simulink model "two_parallel_full_model_simscape"  (R2023b)
settings: Solver=ode1be  StartTime=0.0  StopTime=simlength  FixedStep=ts_sim  MaxStep=ts_sim
undefined symbols (not defined in the file): fclock, fPWM_INV, fPWM_ZVS, gate_nominal_voltage, I_FS, Iout_dc_nom, ki_i_inv, ki_i_zvs, ki_v_inv, ki_v_zvs, kp_i_inv, kp_i_zvs, kp_v_inv, kp_v_zvs, LFi_dc, LFu_ac, magnitude, n10, omega_grid, RCFu_dc, RLFi_dc, RLFu_ac, tc, Tc, tPWM_ZVS, ts_afe, ts_inv, ts_zvs, ugrid_factor, Ugrid_phase_normalization_factor, un_eta_pu, un_xi_pu, up_xi_pu, v1_trafo, v2_trafo, V_FS, Vout_dc_nom
libraries: fl_lib x142, nesl_utility x55, single_phase_transformer_lib x4
(part 2 of 4)

== system two_parallel_full_model_simscape/load/single_phase_ui_measure ==
  Bus Creator : BusCreator  Inputs=2
  Bus Creator1 : BusCreator  Inputs=2
  Current Sensor : fl_lib/Electrical/Electrical Sensors/Current Sensor
  Selector : Selector  InputPortWidth=2  IndexOptions=Index vector (dialog)  Indices=2  OutputSizes=1
  Selector1 : Selector  InputPortWidth=2  IndexOptions=Index vector (dialog)  Indices=1  OutputSizes=1
  To Workspace1 : ToWorkspace  VariableName=load_current_sim  SampleTime=tc
      settings: MaxDataPoints=Nc
  To Workspace2 : ToWorkspace  VariableName=load_voltage_sim  SampleTime=tc
      settings: MaxDataPoints=Nc
  Voltage Sensor : fl_lib/Electrical/Electrical Sensors/Voltage Sensor
  idc/udc zvs modA : Scope  NumInputPorts=2
  iload/imod1/imod2 : Scope  NumInputPorts=2
  iph : nesl_utility/PS-Simulink Converter  PhysicalDomain=network_engine_domain  SubClassName=ps_output  LeftPortType=input  RightPortType=output  PseudoPeriodic=off  Frequencies=[]  VectorFormat=1-D array  Unit=A  AffineConversion=off
  uph : nesl_utility/PS-Simulink Converter  PhysicalDomain=network_engine_domain  SubClassName=ps_output  LeftPortType=input  RightPortType=output  PseudoPeriodic=off  Frequencies=[]  VectorFormat=1-D array  Unit=V  AffineConversion=off
  Ua : PMIOPort  Side=Left
  ua : PMIOPort  Port=2  Side=Right
  Ub : PMIOPort  Port=3  Side=Left
  ub : PMIOPort  Port=4  Side=Right
  tag scope: load_current=global, load_voltage=global
  wires:
  [load_current] -> idc/udc zvs modA/1
  [load_voltage] -> idc/udc zvs modA/2
  Selector1/1 -> [load_current]
  Selector/1 -> [load_voltage]
  Bus Creator/1 -> Selector/1, Selector1/1  "ui_data"
  iph/1 -> Bus Creator/1  "iph"
  uph/1 -> Bus Creator/2  "uph"
  [load_current] -> To Workspace1/1
  [load_voltage] -> To Workspace2/1
  [load_current] -> iload/imod1/imod2/1  "i_load"
  [inverter_current_output_modA] -> Bus Creator1/1  "i_modA"
  [inverter_current_output_modB] -> Bus Creator1/2  "i_modB"
  Bus Creator1/1 -> iload/imod1/imod2/2  "i_modAB"
  connections:
  iph/LConn1 -- Current Sensor/RConn1
  Voltage Sensor/LConn1 -- Current Sensor/LConn1 -- Ua/RConn1
  Current Sensor/RConn2 -- ua/RConn1
  Voltage Sensor/RConn1 -- uph/LConn1
  Voltage Sensor/RConn2 -- Ub/RConn1 -- ub/RConn1

== system two_parallel_full_model_simscape/zvs_modA/dc//dc with galvanic isolation ==
  gate_commands : Inport
  CFu_dc : fl_lib/Electrical/Electrical Elements/Capacitor  c=CFu_dc F  r=RCFu_dc_internal Ohm  g=0 1/Ohm  i_specify=off  i_priority=None  i=0 A  i_nominal_specify=off  i_nominal_unit=A  i_nominal_value=1  v_specify=off  v_priority=None  v=0 V  v_nominal_specify=off  v_nominal_unit=V  v_nominal_value=1  vc_specify=off  vc_priority=High  vc=0 V  vc_nominal_specify=off  vc_nominal_unit=V  vc_nominal_value=1
  Electrical Reference : fl_lib/Electrical/Electrical Elements/Electrical Reference
  RCFu_dc : fl_lib/Electrical/Electrical Elements/Resistor  R=RCFu_dc Ohm  i_specify=off  i_priority=None  i=0 A  i_nominal_specify=off  i_nominal_unit=A  i_nominal_value=1  v_specify=off  v_priority=None  v=0 V  v_nominal_specify=off  v_nominal_unit=V  v_nominal_value=1
  blider1 : fl_lib/Electrical/Electrical Elements/Resistor  R=1e4 Ohm  i_specify=off  i_priority=None  i=0 A  i_nominal_specify=off  i_nominal_unit=A  i_nominal_value=1  v_specify=off  v_priority=None  v=0 V  v_nominal_specify=off  v_nominal_unit=V  v_nominal_value=1
  blider2 : fl_lib/Electrical/Electrical Elements/Resistor  R=1e4 Ohm  i_specify=off  i_priority=None  i=0 A  i_nominal_specify=off  i_nominal_unit=A  i_nominal_value=1  v_specify=off  v_priority=None  v=0 V  v_nominal_specify=off  v_nominal_unit=V  v_nominal_value=1
  stage-1 : Subsystem
      settings: PortSchema="{\"entries\":[{\"content\":{\"sides\":[{\"content\":{\"connectorIds\":[\"LConn1\",\"LConn2\"]},\"type\":\"ConnectorPlacement.EquallySpacedRectSide\",\"uuid\":\"c872503a-61af-4937-bdf2-4de4f8645573\"},{\"content\":{\"connectorIds\":[\"RConn1\",\"RConn2\"],\"side\":\"RIGHT\"},\"type\":\"ConnectorPlacement.EquallySpacedRectSide\",\"uuid\":\"3b83f060-86a2-4569-84b5-d9f7c0485347\"},{\"content\":{\"connectorIds\":[\"In1\"],\"side\":\"TOP\"},\"type\":\"ConnectorPlacement.EquallySpacedRectSide\",\"uuid\":\"bf191d46-ce71-4d15-9dd0-24cc57253577\"}]},\"type\":\"ConnectorPlacement.EquallySpacedConnector\",\"uuid\":\"1b28ceee-25d0-45ae-a3c4-c2563f0d63ba\"}],\"packageUris\":[\"http://schema.mathworks.com/mf0/Connector/R2020b\"],\"version\":\"1.0\"}"
  stage-2 : Subsystem
  Udc(+) : PMIOPort  Side=Left
  udc(+) : PMIOPort  Port=2  Side=Right
  Udc(-) : PMIOPort  Port=3  Side=Left
  udc(-) : PMIOPort  Port=4  Side=Right
  wires:
  gate_commands/1 -> stage-1/1(gate_commands)
  connections:
  stage-2/LConn1 -- stage-1/LConn1
  stage-2/LConn2 -- stage-1/LConn2
  stage-1/RConn1 -- Udc(+)/RConn1
  stage-1/RConn2 -- Udc(-)/RConn1
  CFu_dc/RConn1 -- RCFu_dc/RConn1 -- stage-2/RConn2 -- blider2/RConn1 -- udc(-)/RConn1
  blider2/LConn1 -- blider1/RConn1 -- Electrical Reference/LConn1
  RCFu_dc/LConn1 -- udc(+)/RConn1 -- blider1/LConn1 -- CFu_dc/LConn1 -- stage-2/RConn1

== system two_parallel_full_model_simscape/zvs_modA/grid_rectifier ==
  CFi : fl_lib/Electrical/Electrical Elements/Capacitor  c=CFi_dc F  r=RCFi_dc Ohm  g=0 1/Ohm  i_specify=off  i_priority=None  i=0 A  i_nominal_specify=off  i_nominal_unit=A  i_nominal_value=1  v_specify=off  v_priority=None  v=0 V  v_nominal_specify=off  v_nominal_unit=V  v_nominal_value=1  vc_specify=off  vc_priority=High  vc=0 V  vc_nominal_specify=off  vc_nominal_unit=V  vc_nominal_value=1
  LFi_1 : fl_lib/Electrical/Electrical Elements/Inductor  l=LFi_dc/2 H  r=RLFi_dc/2 Ohm  g=1e-9 1/Ohm  i_specify=on  i_priority=High  i=0 A  i_nominal_specify=off  i_nominal_unit=A  i_nominal_value=1  v_specify=off  v_priority=None  v=0 V  v_nominal_specify=off  v_nominal_unit=V  v_nominal_value=1  i_L_specify=off  i_L_priority=High  i_L=0 A  i_L_nominal_specify=off  i_L_nominal_unit=A  i_L_nominal_value=1
  LFi_2 : fl_lib/Electrical/Electrical Elements/Inductor  l=LFi_dc/2 H  r=RLFi_dc/2 Ohm  g=1e-9 1/Ohm  i_specify=on  i_priority=High  i=0 A  i_nominal_specify=off  i_nominal_unit=A  i_nominal_value=1  v_specify=off  v_priority=None  v=0 V  v_nominal_specify=off  v_nominal_unit=V  v_nominal_value=1  i_L_specify=off  i_L_priority=High  i_L=0 A  i_L_nominal_specify=off  i_L_nominal_unit=A  i_L_nominal_value=1
  three-phase-rectifier : Subsystem
  rectifier_udc(+) : PMIOPort  Side=Right
  ua : PMIOPort  Port=2  Side=Left
  ub : PMIOPort  Port=3  Side=Left
  uc : PMIOPort  Port=4  Side=Left
  rectifier_udc(-) : PMIOPort  Port=5  Side=Right
  connections:
  LFi_1/RConn1 -- rectifier_udc(+)/RConn1 -- CFi/LConn1
  LFi_2/LConn1 -- rectifier_udc(-)/RConn1 -- CFi/RConn1
  LFi_1/LConn1 -- three-phase-rectifier/RConn1
  three-phase-rectifier/LConn1 -- ua/RConn1
  three-phase-rectifier/LConn2 -- ub/RConn1
  three-phase-rectifier/LConn3 -- uc/RConn1
  LFi_2/RConn1 -- three-phase-rectifier/RConn2

== system two_parallel_full_model_simscape/zvs_modA/measurment ==
  To Workspace10 : ToWorkspace  VariableName=vi_CFu_ac_modA_sim  SampleTime=Tc
      settings: MaxDataPoints=Nc
  To Workspace11 : ToWorkspace  VariableName=vi_LFu_ac_modA_sim  SampleTime=Tc
      settings: MaxDataPoints=Nc
  To Workspace12 : ToWorkspace  VariableName=vi_LFi_dc_modA_sim  SampleTime=Tc
      settings: MaxDataPoints=Nc
  To Workspace13 : ToWorkspace  VariableName=vi_Ls_modA_sim  SampleTime=Tc
      settings: MaxDataPoints=Nc
  To Workspace14 : ToWorkspace  VariableName=vi_CFi_dc_modA_sim  SampleTime=Tc
      settings: MaxDataPoints=Nc
  To Workspace15 : ToWorkspace  VariableName=i_d_rect_modA_sim  SampleTime=Tc
      settings: MaxDataPoints=Nc
  To Workspace2 : ToWorkspace  VariableName=vi_RCFu_dc_modA_sim  SampleTime=Tc
      settings: MaxDataPoints=Nc
  To Workspace3 : ToWorkspace  VariableName=vi_LFu_dc_modA_sim  SampleTime=Tc
      settings: MaxDataPoints=Nc
  To Workspace4 : ToWorkspace  VariableName=vi_Cs_modA_sim  SampleTime=Tc
      settings: MaxDataPoints=Nc
  To Workspace5 : ToWorkspace  VariableName=vi_load_modA_sim  SampleTime=Tc
      settings: MaxDataPoints=Nc
  To Workspace6 : ToWorkspace  VariableName=vi_CFu_dc_modA_sim  SampleTime=Tc
      settings: MaxDataPoints=Nc
  To Workspace7 : ToWorkspace  VariableName=vdc_in_modA_sim  SampleTime=Tc
      settings: MaxDataPoints=Nc
  To Workspace8 : ToWorkspace  VariableName=Isnubber_H_modA_sim  SampleTime=Tc
      settings: MaxDataPoints=Nc
  To Workspace9 : ToWorkspace  VariableName=Isnubber_Rect1_modA_sim  SampleTime=Tc
      settings: MaxDataPoints=Nc

== system two_parallel_full_model_simscape/zvs_modA/single_phase_ui_measure ==
  Bus Creator : BusCreator  Inputs=2
  Current Sensor : fl_lib/Electrical/Electrical Sensors/Current Sensor
  Selector : Selector  InputPortWidth=2  IndexOptions=Index vector (dialog)  Indices=2  OutputSizes=1
  Selector1 : Selector  InputPortWidth=2  IndexOptions=Index vector (dialog)  Indices=1  OutputSizes=1
  To Workspace1 : ToWorkspace  VariableName=zvs_current_output_modA_sim  SampleTime=tc
      settings: MaxDataPoints=Nc
  To Workspace2 : ToWorkspace  VariableName=zvs_voltage_output_modA_sim  SampleTime=tc
      settings: MaxDataPoints=Nc
  Voltage Sensor : fl_lib/Electrical/Electrical Sensors/Voltage Sensor
  idc/udc zvs modA : Scope  NumInputPorts=2
  iph : nesl_utility/PS-Simulink Converter  PhysicalDomain=network_engine_domain  SubClassName=ps_output  LeftPortType=input  RightPortType=output  PseudoPeriodic=off  Frequencies=[]  VectorFormat=1-D array  Unit=A  AffineConversion=off
  uph : nesl_utility/PS-Simulink Converter  PhysicalDomain=network_engine_domain  SubClassName=ps_output  LeftPortType=input  RightPortType=output  PseudoPeriodic=off  Frequencies=[]  VectorFormat=1-D array  Unit=V  AffineConversion=off
  Udc(+) : PMIOPort  Side=Left
  udc(+) : PMIOPort  Port=2  Side=Right
  Udc(-) : PMIOPort  Port=3  Side=Left
  udc(-) : PMIOPort  Port=4  Side=Right
  tag scope: zvs_current_output_modA=global, zvs_voltage_output_modA=global
  wires:
  [zvs_current_output_modA] -> idc/udc zvs modA/1  "zvs_current_output_modA"
  [zvs_voltage_output_modA] -> idc/udc zvs modA/2  "zvs_voltage_output_modA"
  Selector1/1 -> [zvs_current_output_modA]
  Selector/1 -> [zvs_voltage_output_modA]
  Bus Creator/1 -> Selector/1, Selector1/1  "ui_data"
  iph/1 -> Bus Creator/1  "iph"
  uph/1 -> Bus Creator/2  "uph"
  [zvs_current_output_modA] -> To Workspace1/1
  [zvs_voltage_output_modA] -> To Workspace2/1
  connections:
  iph/LConn1 -- Current Sensor/RConn1
  Voltage Sensor/LConn1 -- Current Sensor/LConn1 -- Udc(+)/RConn1
  Current Sensor/RConn2 -- udc(+)/RConn1
  Voltage Sensor/RConn1 -- uph/LConn1
  Voltage Sensor/RConn2 -- Udc(-)/RConn1 -- udc(-)/RConn1

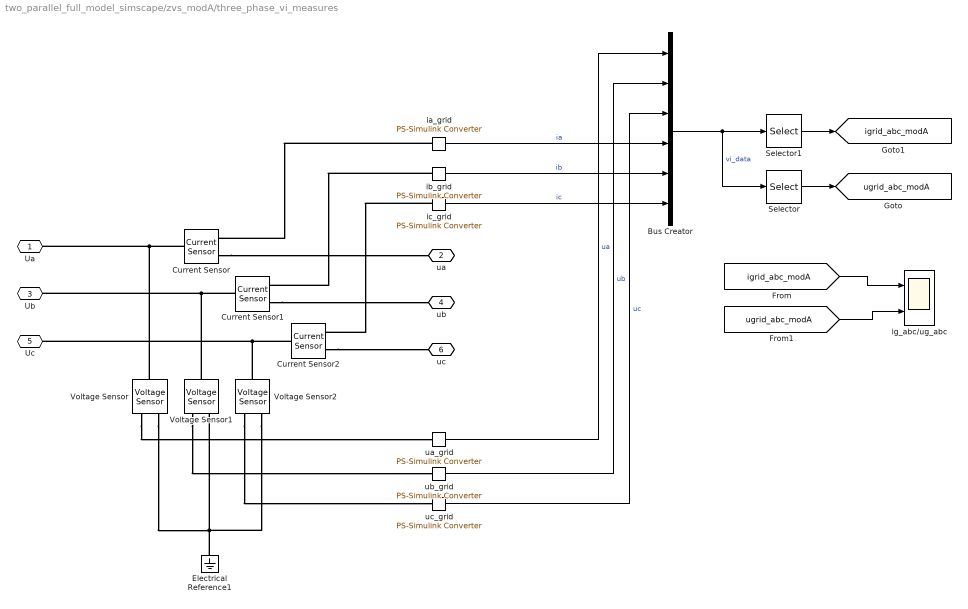
== system two_parallel_full_model_simscape/zvs_modA/three_phase_vi_measures ==
  Bus Creator : BusCreator  Inputs=6
  Current Sensor : fl_lib/Electrical/Electrical Sensors/Current Sensor
  Current Sensor1 : fl_lib/Electrical/Electrical Sensors/Current Sensor
  Current Sensor2 : fl_lib/Electrical/Electrical Sensors/Current Sensor
  Electrical Reference1 : fl_lib/Electrical/Electrical Elements/Electrical Reference
  Selector : Selector  InputPortWidth=6  IndexOptions=Index vector (dialog)  Indices=[1 2 3]  OutputSizes=1
  Selector1 : Selector  InputPortWidth=6  IndexOptions=Index vector (dialog)  Indices=[4 5 6]  OutputSizes=1
  Voltage Sensor : fl_lib/Electrical/Electrical Sensors/Voltage Sensor
  Voltage Sensor1 : fl_lib/Electrical/Electrical Sensors/Voltage Sensor
  Voltage Sensor2 : fl_lib/Electrical/Electrical Sensors/Voltage Sensor
  ia_grid : nesl_utility/PS-Simulink Converter  PhysicalDomain=network_engine_domain  SubClassName=ps_output  LeftPortType=input  RightPortType=output  PseudoPeriodic=off  Frequencies=[]  VectorFormat=1-D array  Unit=A  AffineConversion=off
  ib_grid : nesl_utility/PS-Simulink Converter  PhysicalDomain=network_engine_domain  SubClassName=ps_output  LeftPortType=input  RightPortType=output  PseudoPeriodic=off  Frequencies=[]  VectorFormat=1-D array  Unit=A  AffineConversion=off
  ic_grid : nesl_utility/PS-Simulink Converter  PhysicalDomain=network_engine_domain  SubClassName=ps_output  LeftPortType=input  RightPortType=output  PseudoPeriodic=off  Frequencies=[]  VectorFormat=1-D array  Unit=A  AffineConversion=off
  ig_abc/ug_abc : Scope  NumInputPorts=2
  ua_grid : nesl_utility/PS-Simulink Converter  PhysicalDomain=network_engine_domain  SubClassName=ps_output  LeftPortType=input  RightPortType=output  PseudoPeriodic=off  Frequencies=[]  VectorFormat=1-D array  Unit=V  AffineConversion=off
  ub_grid : nesl_utility/PS-Simulink Converter  PhysicalDomain=network_engine_domain  SubClassName=ps_output  LeftPortType=input  RightPortType=output  PseudoPeriodic=off  Frequencies=[]  VectorFormat=1-D array  Unit=V  AffineConversion=off
  uc_grid : nesl_utility/PS-Simulink Converter  PhysicalDomain=network_engine_domain  SubClassName=ps_output  LeftPortType=input  RightPortType=output  PseudoPeriodic=off  Frequencies=[]  VectorFormat=1-D array  Unit=V  AffineConversion=off
  Ua : PMIOPort  Side=Left
  ua : PMIOPort  Port=2  Side=Right
  Ub : PMIOPort  Port=3  Side=Left
  ub : PMIOPort  Port=4  Side=Right
  Uc : PMIOPort  Port=5  Side=Left
  uc : PMIOPort  Port=6  Side=Right
  tag scope: igrid_abc_modA=global, ugrid_abc_modA=global
  wires:
  Bus Creator/1 -> Selector1/1, Selector/1  "vi_data"
  Selector/1 -> [ugrid_abc_modA]
  ib_grid/1 -> Bus Creator/5  "ib"
  ia_grid/1 -> Bus Creator/4  "ia"
  ic_grid/1 -> Bus Creator/6  "ic"
  ua_grid/1 -> Bus Creator/1  "ua"
  ub_grid/1 -> Bus Creator/2  "ub"
  uc_grid/1 -> Bus Creator/3  "uc"
  Selector1/1 -> [igrid_abc_modA]
  [ugrid_abc_modA] -> ig_abc/ug_abc/2
  [igrid_abc_modA] -> ig_abc/ug_abc/1
  connections:
  Current Sensor1/LConn1 -- Ub/RConn1 -- Voltage Sensor1/LConn1
  Electrical Reference1/LConn1 -- Voltage Sensor/RConn2 -- Voltage Sensor2/RConn2 -- Voltage Sensor1/RConn2
  Voltage Sensor/RConn1 -- ua_grid/LConn1
  Current Sensor/RConn2 -- ua/RConn1
  Voltage Sensor1/RConn1 -- ub_grid/LConn1
  Voltage Sensor2/LConn1 -- Current Sensor2/LConn1 -- Uc/RConn1
  Current Sensor/LConn1 -- Ua/RConn1 -- Voltage Sensor/LConn1
  Current Sensor1/RConn2 -- ub/RConn1
  Voltage Sensor2/RConn1 -- uc_grid/LConn1
  ib_grid/LConn1 -- Current Sensor1/RConn1
  ia_grid/LConn1 -- Current Sensor/RConn1
  ic_grid/LConn1 -- Current Sensor2/RConn1
  Current Sensor2/RConn2 -- uc/RConn1

== system two_parallel_full_model_simscape/zvs_modA/zvs_ctrl ==
  Bus Creator : BusCreator  Inputs=4
  modulator : Subsystem
  references : Subsystem
  sampling_i_filter1 : Subsystem
  sampling_v_filter1 : Subsystem
  sampling_v_filter2 : Subsystem
  vi ctrl : Subsystem
  gate_commands : Outport
  wires:
  [zvs_voltage_output_modA] -> sampling_v_filter1/1(in)
  [zvs_current_output_modA] -> sampling_i_filter1/1(in)
  vi ctrl/1(phase_displacement) -> modulator/1(phase_displacement)
  sampling_i_filter1/1(out_pu) -> vi ctrl/1(iout)
  sampling_v_filter1/1(out_pu) -> vi ctrl/2(vout)
  sampling_v_filter2/1(out_pu) -> vi ctrl/3(vout_ref)
  references/1(vout_ref) -> sampling_v_filter2/1(in)
  Bus Creator/1 -> gate_commands/1
  modulator/1(gate_Q1) -> Bus Creator/1
  modulator/2(gate_Q2) -> Bus Creator/2
  modulator/3(gate_Q3) -> Bus Creator/3
  modulator/4(gate_Q4) -> Bus Creator/4

== system two_parallel_full_model_simscape/zvs_modB/dc//dc with galvanic isolation ==
  gate_commands : Inport
  CFu_dc : fl_lib/Electrical/Electrical Elements/Capacitor  c=CFu_dc F  r=RCFu_dc_internal Ohm  g=0 1/Ohm  i_specify=off  i_priority=None  i=0 A  i_nominal_specify=off  i_nominal_unit=A  i_nominal_value=1  v_specify=off  v_priority=None  v=0 V  v_nominal_specify=off  v_nominal_unit=V  v_nominal_value=1  vc_specify=off  vc_priority=High  vc=0 V  vc_nominal_specify=off  vc_nominal_unit=V  vc_nominal_value=1
  Electrical Reference : fl_lib/Electrical/Electrical Elements/Electrical Reference
  RCFu_dc : fl_lib/Electrical/Electrical Elements/Resistor  R=RCFu_dc Ohm  i_specify=off  i_priority=None  i=0 A  i_nominal_specify=off  i_nominal_unit=A  i_nominal_value=1  v_specify=off  v_priority=None  v=0 V  v_nominal_specify=off  v_nominal_unit=V  v_nominal_value=1
  blider1 : fl_lib/Electrical/Electrical Elements/Resistor  R=1e4 Ohm  i_specify=off  i_priority=None  i=0 A  i_nominal_specify=off  i_nominal_unit=A  i_nominal_value=1  v_specify=off  v_priority=None  v=0 V  v_nominal_specify=off  v_nominal_unit=V  v_nominal_value=1
  blider2 : fl_lib/Electrical/Electrical Elements/Resistor  R=1e4 Ohm  i_specify=off  i_priority=None  i=0 A  i_nominal_specify=off  i_nominal_unit=A  i_nominal_value=1  v_specify=off  v_priority=None  v=0 V  v_nominal_specify=off  v_nominal_unit=V  v_nominal_value=1
  stage-1 : Subsystem
      settings: PortSchema="{\"entries\":[{\"content\":{\"sides\":[{\"content\":{\"connectorIds\":[\"LConn1\",\"LConn2\"]},\"type\":\"ConnectorPlacement.EquallySpacedRectSide\",\"uuid\":\"c872503a-61af-4937-bdf2-4de4f8645573\"},{\"content\":{\"connectorIds\":[\"RConn1\",\"RConn2\"],\"side\":\"RIGHT\"},\"type\":\"ConnectorPlacement.EquallySpacedRectSide\",\"uuid\":\"3b83f060-86a2-4569-84b5-d9f7c0485347\"},{\"content\":{\"connectorIds\":[\"In1\"],\"side\":\"TOP\"},\"type\":\"ConnectorPlacement.EquallySpacedRectSide\",\"uuid\":\"bf191d46-ce71-4d15-9dd0-24cc57253577\"}]},\"type\":\"ConnectorPlacement.EquallySpacedConnector\",\"uuid\":\"1b28ceee-25d0-45ae-a3c4-c2563f0d63ba\"}],\"packageUris\":[\"http://schema.mathworks.com/mf0/Connector/R2020b\"],\"version\":\"1.0\"}"
  stage-2 : Subsystem
  Udc(+) : PMIOPort  Side=Left
  udc(+) : PMIOPort  Port=2  Side=Right
  Udc(-) : PMIOPort  Port=3  Side=Left
  udc(-) : PMIOPort  Port=4  Side=Right
  wires:
  gate_commands/1 -> stage-1/1(gate_commands)
  connections:
  stage-2/RConn1 -- CFu_dc/LConn1 -- blider1/LConn1 -- udc(+)/RConn1 -- RCFu_dc/LConn1
  Electrical Reference/LConn1 -- blider1/RConn1 -- blider2/LConn1
  udc(-)/RConn1 -- blider2/RConn1 -- stage-2/RConn2 -- RCFu_dc/RConn1 -- CFu_dc/RConn1
  stage-1/RConn2 -- Udc(-)/RConn1
  stage-1/RConn1 -- Udc(+)/RConn1
  stage-2/LConn2 -- stage-1/LConn2
  stage-2/LConn1 -- stage-1/LConn1

== system two_parallel_full_model_simscape/zvs_modB/grid_rectifier ==
  CFi : fl_lib/Electrical/Electrical Elements/Capacitor  c=CFi_dc F  r=RCFi_dc Ohm  g=0 1/Ohm  i_specify=off  i_priority=None  i=0 A  i_nominal_specify=off  i_nominal_unit=A  i_nominal_value=1  v_specify=off  v_priority=None  v=0 V  v_nominal_specify=off  v_nominal_unit=V  v_nominal_value=1  vc_specify=off  vc_priority=High  vc=0 V  vc_nominal_specify=off  vc_nominal_unit=V  vc_nominal_value=1
  LFi_1 : fl_lib/Electrical/Electrical Elements/Inductor  l=LFi_dc/2 H  r=RLFi_dc/2 Ohm  g=1e-9 1/Ohm  i_specify=on  i_priority=High  i=0 A  i_nominal_specify=off  i_nominal_unit=A  i_nominal_value=1  v_specify=off  v_priority=None  v=0 V  v_nominal_specify=off  v_nominal_unit=V  v_nominal_value=1  i_L_specify=off  i_L_priority=High  i_L=0 A  i_L_nominal_specify=off  i_L_nominal_unit=A  i_L_nominal_value=1
  LFi_2 : fl_lib/Electrical/Electrical Elements/Inductor  l=LFi_dc/2 H  r=RLFi_dc/2 Ohm  g=1e-9 1/Ohm  i_specify=on  i_priority=High  i=0 A  i_nominal_specify=off  i_nominal_unit=A  i_nominal_value=1  v_specify=off  v_priority=None  v=0 V  v_nominal_specify=off  v_nominal_unit=V  v_nominal_value=1  i_L_specify=off  i_L_priority=High  i_L=0 A  i_L_nominal_specify=off  i_L_nominal_unit=A  i_L_nominal_value=1
  three-phase-rectifier : Subsystem
  rectifier_udc(+) : PMIOPort  Side=Right
  ua : PMIOPort  Port=2  Side=Left
  ub : PMIOPort  Port=3  Side=Left
  uc : PMIOPort  Port=4  Side=Left
  rectifier_udc(-) : PMIOPort  Port=5  Side=Right
  connections:
  LFi_2/RConn1 -- three-phase-rectifier/RConn2
  three-phase-rectifier/LConn3 -- uc/RConn1
  three-phase-rectifier/LConn2 -- ub/RConn1
  three-phase-rectifier/LConn1 -- ua/RConn1
  LFi_1/LConn1 -- three-phase-rectifier/RConn1
  CFi/RConn1 -- rectifier_udc(-)/RConn1 -- LFi_2/LConn1
  CFi/LConn1 -- rectifier_udc(+)/RConn1 -- LFi_1/RConn1

== system two_parallel_full_model_simscape/zvs_modB/measurment ==
  To Workspace10 : ToWorkspace  VariableName=vi_CFu_ac_modA_sim  SampleTime=Tc
      settings: MaxDataPoints=Nc
  To Workspace11 : ToWorkspace  VariableName=vi_LFu_ac_modA_sim  SampleTime=Tc
      settings: MaxDataPoints=Nc
  To Workspace12 : ToWorkspace  VariableName=vi_LFi_dc_modA_sim  SampleTime=Tc
      settings: MaxDataPoints=Nc
  To Workspace13 : ToWorkspace  VariableName=vi_Ls_modA_sim  SampleTime=Tc
      settings: MaxDataPoints=Nc
  To Workspace14 : ToWorkspace  VariableName=vi_CFi_dc_modA_sim  SampleTime=Tc
      settings: MaxDataPoints=Nc
  To Workspace15 : ToWorkspace  VariableName=i_d_rect_modA_sim  SampleTime=Tc
      settings: MaxDataPoints=Nc
  To Workspace2 : ToWorkspace  VariableName=vi_RCFu_dc_modA_sim  SampleTime=Tc
      settings: MaxDataPoints=Nc
  To Workspace3 : ToWorkspace  VariableName=vi_LFu_dc_modA_sim  SampleTime=Tc
      settings: MaxDataPoints=Nc
  To Workspace4 : ToWorkspace  VariableName=vi_Cs_modA_sim  SampleTime=Tc
      settings: MaxDataPoints=Nc
  To Workspace5 : ToWorkspace  VariableName=vi_load_modA_sim  SampleTime=Tc
      settings: MaxDataPoints=Nc
  To Workspace6 : ToWorkspace  VariableName=vi_CFu_dc_modA_sim  SampleTime=Tc
      settings: MaxDataPoints=Nc
  To Workspace7 : ToWorkspace  VariableName=vdc_in_modA_sim  SampleTime=Tc
      settings: MaxDataPoints=Nc
  To Workspace8 : ToWorkspace  VariableName=Isnubber_H_modA_sim  SampleTime=Tc
      settings: MaxDataPoints=Nc
  To Workspace9 : ToWorkspace  VariableName=Isnubber_Rect1_modA_sim  SampleTime=Tc
      settings: MaxDataPoints=Nc

== system two_parallel_full_model_simscape/zvs_modB/single_phase_ui_measure ==
  Bus Creator : BusCreator  Inputs=2
  Current Sensor : fl_lib/Electrical/Electrical Sensors/Current Sensor
  Selector : Selector  InputPortWidth=2  IndexOptions=Index vector (dialog)  Indices=2  OutputSizes=1
  Selector1 : Selector  InputPortWidth=2  IndexOptions=Index vector (dialog)  Indices=1  OutputSizes=1
  To Workspace1 : ToWorkspace  VariableName=zvs_current_output_modB_sim  SampleTime=tc
      settings: MaxDataPoints=Nc
  To Workspace2 : ToWorkspace  VariableName=zvs_voltage_output_modB_sim  SampleTime=tc
      settings: MaxDataPoints=Nc
  Voltage Sensor : fl_lib/Electrical/Electrical Sensors/Voltage Sensor
  idc/udc zvs modB : Scope  NumInputPorts=2
  iph : nesl_utility/PS-Simulink Converter  PhysicalDomain=network_engine_domain  SubClassName=ps_output  LeftPortType=input  RightPortType=output  PseudoPeriodic=off  Frequencies=[]  VectorFormat=1-D array  Unit=A  AffineConversion=off
  uph : nesl_utility/PS-Simulink Converter  PhysicalDomain=network_engine_domain  SubClassName=ps_output  LeftPortType=input  RightPortType=output  PseudoPeriodic=off  Frequencies=[]  VectorFormat=1-D array  Unit=V  AffineConversion=off
  Udc(+) : PMIOPort  Side=Left
  udc(+) : PMIOPort  Port=2  Side=Right
  Udc(-) : PMIOPort  Port=3  Side=Left
  udc(-) : PMIOPort  Port=4  Side=Right
  tag scope: zvs_current_output_modB=global, zvs_voltage_output_modB=global
  wires:
  [zvs_voltage_output_modB] -> To Workspace2/1
  [zvs_current_output_modB] -> To Workspace1/1
  uph/1 -> Bus Creator/2  "uph"
  iph/1 -> Bus Creator/1  "iph"
  Bus Creator/1 -> Selector1/1, Selector/1  "ui_data"
  Selector/1 -> [zvs_voltage_output_modB]
  Selector1/1 -> [zvs_current_output_modB]
  [zvs_voltage_output_modB] -> idc/udc zvs modB/2  "zvs_voltage_output_modB"
  [zvs_current_output_modB] -> idc/udc zvs modB/1  "zvs_current_output_modB"
  connections:
  udc(-)/RConn1 -- Udc(-)/RConn1 -- Voltage Sensor/RConn2
  Voltage Sensor/RConn1 -- uph/LConn1
  Current Sensor/RConn2 -- udc(+)/RConn1
  Udc(+)/RConn1 -- Current Sensor/LConn1 -- Voltage Sensor/LConn1
  iph/LConn1 -- Current Sensor/RConn1

== system two_parallel_full_model_simscape/zvs_modB/three_phase_vi_measures ==
  Bus Creator : BusCreator  Inputs=6
  Current Sensor : fl_lib/Electrical/Electrical Sensors/Current Sensor
  Current Sensor1 : fl_lib/Electrical/Electrical Sensors/Current Sensor
  Current Sensor2 : fl_lib/Electrical/Electrical Sensors/Current Sensor
  Electrical Reference1 : fl_lib/Electrical/Electrical Elements/Electrical Reference
  Selector : Selector  InputPortWidth=6  IndexOptions=Index vector (dialog)  Indices=[1 2 3]  OutputSizes=1
  Selector1 : Selector  InputPortWidth=6  IndexOptions=Index vector (dialog)  Indices=[4 5 6]  OutputSizes=1
  Voltage Sensor : fl_lib/Electrical/Electrical Sensors/Voltage Sensor
  Voltage Sensor1 : fl_lib/Electrical/Electrical Sensors/Voltage Sensor
  Voltage Sensor2 : fl_lib/Electrical/Electrical Sensors/Voltage Sensor
  ia_grid : nesl_utility/PS-Simulink Converter  PhysicalDomain=network_engine_domain  SubClassName=ps_output  LeftPortType=input  RightPortType=output  PseudoPeriodic=off  Frequencies=[]  VectorFormat=1-D array  Unit=A  AffineConversion=off
  ib_grid : nesl_utility/PS-Simulink Converter  PhysicalDomain=network_engine_domain  SubClassName=ps_output  LeftPortType=input  RightPortType=output  PseudoPeriodic=off  Frequencies=[]  VectorFormat=1-D array  Unit=A  AffineConversion=off
  ic_grid : nesl_utility/PS-Simulink Converter  PhysicalDomain=network_engine_domain  SubClassName=ps_output  LeftPortType=input  RightPortType=output  PseudoPeriodic=off  Frequencies=[]  VectorFormat=1-D array  Unit=A  AffineConversion=off
  ig_abc/ug_abc : Scope  NumInputPorts=2
  ua_grid : nesl_utility/PS-Simulink Converter  PhysicalDomain=network_engine_domain  SubClassName=ps_output  LeftPortType=input  RightPortType=output  PseudoPeriodic=off  Frequencies=[]  VectorFormat=1-D array  Unit=V  AffineConversion=off
  ub_grid : nesl_utility/PS-Simulink Converter  PhysicalDomain=network_engine_domain  SubClassName=ps_output  LeftPortType=input  RightPortType=output  PseudoPeriodic=off  Frequencies=[]  VectorFormat=1-D array  Unit=V  AffineConversion=off
  uc_grid : nesl_utility/PS-Simulink Converter  PhysicalDomain=network_engine_domain  SubClassName=ps_output  LeftPortType=input  RightPortType=output  PseudoPeriodic=off  Frequencies=[]  VectorFormat=1-D array  Unit=V  AffineConversion=off
  Ua : PMIOPort  Side=Left
  ua : PMIOPort  Port=2  Side=Right
  Ub : PMIOPort  Port=3  Side=Left
  ub : PMIOPort  Port=4  Side=Right
  Uc : PMIOPort  Port=5  Side=Left
  uc : PMIOPort  Port=6  Side=Right
  tag scope: igrid_abc_modB=global, ugrid_abc_modB=global
  wires:
  [igrid_abc_modB] -> ig_abc/ug_abc/1
  [ugrid_abc_modB] -> ig_abc/ug_abc/2
  Selector1/1 -> [igrid_abc_modB]
  uc_grid/1 -> Bus Creator/3  "uc"
  ub_grid/1 -> Bus Creator/2  "ub"
  ua_grid/1 -> Bus Creator/1  "ua"
  ic_grid/1 -> Bus Creator/6  "ic"
  ia_grid/1 -> Bus Creator/4  "ia"
  ib_grid/1 -> Bus Creator/5  "ib"
  Selector/1 -> [ugrid_abc_modB]
  Bus Creator/1 -> Selector/1, Selector1/1  "vi_data"
  connections:
  Current Sensor2/RConn2 -- uc/RConn1
  ic_grid/LConn1 -- Current Sensor2/RConn1
  ia_grid/LConn1 -- Current Sensor/RConn1
  ib_grid/LConn1 -- Current Sensor1/RConn1
  Voltage Sensor2/RConn1 -- uc_grid/LConn1
  Current Sensor1/RConn2 -- ub/RConn1
  Voltage Sensor/LConn1 -- Ua/RConn1 -- Current Sensor/LConn1
  Uc/RConn1 -- Current Sensor2/LConn1 -- Voltage Sensor2/LConn1
  Voltage Sensor1/RConn1 -- ub_grid/LConn1
  Current Sensor/RConn2 -- ua/RConn1
  Voltage Sensor/RConn1 -- ua_grid/LConn1
  Voltage Sensor1/RConn2 -- Voltage Sensor2/RConn2 -- Voltage Sensor/RConn2 -- Electrical Reference1/LConn1
  Voltage Sensor1/LConn1 -- Ub/RConn1 -- Current Sensor1/LConn1

== system two_parallel_full_model_simscape/zvs_modB/zvs_ctrl ==
  Bus Creator : BusCreator  Inputs=4
  modulator : Subsystem
  references : Subsystem
  sampling_i_filter1 : Subsystem
  sampling_v_filter1 : Subsystem
  sampling_v_filter2 : Subsystem
  vi ctrl : Subsystem
  gate_commands : Outport
  wires:
  modulator/4(gate_Q4) -> Bus Creator/4
  modulator/3(gate_Q3) -> Bus Creator/3
  modulator/2(gate_Q2) -> Bus Creator/2
  modulator/1(gate_Q1) -> Bus Creator/1
  Bus Creator/1 -> gate_commands/1
  references/1(vout_ref) -> sampling_v_filter2/1(in)
  sampling_v_filter2/1(out_pu) -> vi ctrl/3(vout_ref)
  sampling_v_filter1/1(out_pu) -> vi ctrl/2(vout)
  sampling_i_filter1/1(out_pu) -> vi ctrl/1(iout)
  vi ctrl/1(phase_displacement) -> modulator/1(phase_displacement)
  [zvs_current_output_modB] -> sampling_i_filter1/1(in)
  [zvs_voltage_output_modB] -> sampling_v_filter1/1(in)

== system two_parallel_full_model_simscape/grid/grid_emulator/grid_source ==
  phase_gen : Subsystem
  voltage_grid : Subsystem
  voltage_source : Subsystem
  ur_grid : Outport
  us_grid : Outport  Port=2
  ut_grid : Outport  Port=3
  wires:
  phase_gen/1(grid_emu_phase) -> voltage_grid/1(grid_emu_phase)  "grid_emu_phase"
  voltage_source/2(vn_xi) -> voltage_grid/3(Vxi_n)
  voltage_source/1(vp_xi) -> voltage_grid/2(Vxi_p)
  voltage_source/3(vn_eta) -> voltage_grid/4(Veta_n)
  voltage_grid/3(ut_grid) -> ut_grid/1
  voltage_grid/1(ur_grid) -> ur_grid/1
  voltage_grid/2(us_grid) -> us_grid/1

== system two_parallel_full_model_simscape/grid/instantaneus_power/abc2alphabeta ==
  a : Inport
  b : Inport  Port=2
  c : Inport  Port=3
  abc2alphabeta : Subsystem
  vline_alpha : Outport  VectorParamsAs1DForOutWhenUnconnected=off
  vline_beta : Outport  Port=2  VectorParamsAs1DForOutWhenUnconnected=off
  wires:
  a/1 -> abc2alphabeta/1(a)
  b/1 -> abc2alphabeta/2(b)
  c/1 -> abc2alphabeta/3(c)
  abc2alphabeta/2("beta ") -> vline_beta/1
  abc2alphabeta/1("alpha ") -> vline_alpha/1

== system two_parallel_full_model_simscape/grid/instantaneus_power/abc2alphabeta  ==
  a : Inport
  b : Inport  Port=2
  c : Inport  Port=3
  abc->alphabeta : Subsystem
  i_line_alpha : Outport  VectorParamsAs1DForOutWhenUnconnected=off
  i_line_beta : Outport  Port=2  VectorParamsAs1DForOutWhenUnconnected=off
  wires:
  abc->alphabeta/1("alpha ") -> i_line_alpha/1
  abc->alphabeta/2("beta ") -> i_line_beta/1
  c/1 -> abc->alphabeta/3(c)
  b/1 -> abc->alphabeta/2(b)
  a/1 -> abc->alphabeta/1(a)

== system two_parallel_full_model_simscape/grid/instantaneus_power/moving_avarage ==
  In : Inport
  Gain1 : Gain  Gain=omega_grid/2/pi  SaturateOnIntegerOverflow=on  OutDataTypeStr=Inherit: Same as input  ParamDataTypeStr=Inherit: Same as input
  Sum4 : Sum  SaturateOnIntegerOverflow=on
  Sum8 : Sum  Inputs=+-  InputSameDT=on  SaturateOnIntegerOverflow=on  OutDataTypeStr=Inherit: Same as first input
  Transport Delay : TransportDelay  DelayTime=2*pi/omega_grid  BufferSize=2048*4  PadeOrder=2
  Unit Delay2 : UnitDelay  SampleTime=ts_afe  HasFrameUpgradeWarning=on
  kp2 : Gain  Gain=ts_afe  SaturateOnIntegerOverflow=on  OutDataTypeStr=Inherit: Same as input  ParamDataTypeStr=Inherit: Same as input
  Mean : Outport  VectorParamsAs1DForOutWhenUnconnected=off
  wires:
  Transport Delay/1 -> Sum8/2
  Sum4/1 -> Sum8/1, Transport Delay/1, Unit Delay2/1
  Sum8/1 -> Gain1/1
  In/1 -> kp2/1
  Unit Delay2/1 -> Sum4/2
  kp2/1 -> Sum4/1
  Gain1/1 -> Mean/1

== system two_parallel_full_model_simscape/grid/instantaneus_power/moving_avarage1 ==
  In : Inport
  Gain1 : Gain  Gain=omega_grid/2/pi  SaturateOnIntegerOverflow=on  OutDataTypeStr=Inherit: Same as input  ParamDataTypeStr=Inherit: Same as input
  Sum4 : Sum  SaturateOnIntegerOverflow=on
  Sum8 : Sum  Inputs=+-  InputSameDT=on  SaturateOnIntegerOverflow=on  OutDataTypeStr=Inherit: Same as first input
  Transport Delay : TransportDelay  DelayTime=2*pi/omega_grid  BufferSize=2048*4  PadeOrder=2
  Unit Delay2 : UnitDelay  SampleTime=ts_afe  HasFrameUpgradeWarning=on
  kp2 : Gain  Gain=ts_afe  SaturateOnIntegerOverflow=on  OutDataTypeStr=Inherit: Same as input  ParamDataTypeStr=Inherit: Same as input
  Mean : Outport  VectorParamsAs1DForOutWhenUnconnected=off
  wires:
  Gain1/1 -> Mean/1
  kp2/1 -> Sum4/1
  Unit Delay2/1 -> Sum4/2
  In/1 -> kp2/1
  Sum8/1 -> Gain1/1
  Sum4/1 -> Unit Delay2/1, Transport Delay/1, Sum8/1
  Transport Delay/1 -> Sum8/2

== system two_parallel_full_model_simscape/grid/instantaneus_power/rms ==
  In1 : Inport
  Gain : Gain  Gain=n10-1
  Gain1 : Gain  Gain=1/n10
  Math Function : Math  Operator=magnitude^2  SignedPower=on
  Sqrt : Sqrt
  Sum : Sum  Inputs=|++
  Unit Delay : UnitDelay  SampleTime=ts_afe  HasFrameUpgradeWarning=on
  Out1 : Outport  VectorParamsAs1DForOutWhenUnconnected=off
  wires:
  In1/1 -> Math Function/1
  Sum/1 -> Gain1/1
  Gain1/1 -> Sqrt/1, Unit Delay/1
  Unit Delay/1 -> Gain/1
  Math Function/1 -> Sum/1
  Sqrt/1 -> Out1/1
  Gain/1 -> Sum/2

== system two_parallel_full_model_simscape/grid/instantaneus_power/rms1 ==
  In1 : Inport
  Gain : Gain  Gain=n10-1
  Gain1 : Gain  Gain=1/n10
  Math Function : Math  Operator=magnitude^2  SignedPower=on
  Sqrt : Sqrt
  Sum : Sum  Inputs=|++
  Unit Delay : UnitDelay  SampleTime=ts_afe  HasFrameUpgradeWarning=on
  Out1 : Outport  VectorParamsAs1DForOutWhenUnconnected=off
  wires:
  Gain/1 -> Sum/2
  Sqrt/1 -> Out1/1
  Math Function/1 -> Sum/1
  Unit Delay/1 -> Gain/1
  Gain1/1 -> Unit Delay/1, Sqrt/1
  Sum/1 -> Gain1/1
  In1/1 -> Math Function/1

== system two_parallel_full_model_simscape/grid/instantaneus_power/rms2 ==
  In1 : Inport
  Gain : Gain  Gain=n10-1
  Gain1 : Gain  Gain=1/n10
  Math Function : Math  Operator=magnitude^2  SignedPower=on
  Sqrt : Sqrt
  Sum : Sum  Inputs=|++
  Unit Delay : UnitDelay  SampleTime=ts_afe  HasFrameUpgradeWarning=on
  Out1 : Outport  VectorParamsAs1DForOutWhenUnconnected=off
  wires:
  In1/1 -> Math Function/1
  Sum/1 -> Gain1/1
  Gain1/1 -> Sqrt/1, Unit Delay/1
  Unit Delay/1 -> Gain/1
  Math Function/1 -> Sum/1
  Sqrt/1 -> Out1/1
  Gain/1 -> Sum/2

== system two_parallel_full_model_simscape/grid/instantaneus_power/rms3 ==
  In1 : Inport
  Gain : Gain  Gain=n10-1
  Gain1 : Gain  Gain=1/n10
  Math Function : Math  Operator=magnitude^2  SignedPower=on
  Sqrt : Sqrt
  Sum : Sum  Inputs=|++
  Unit Delay : UnitDelay  SampleTime=ts_afe  HasFrameUpgradeWarning=on
  Out1 : Outport  VectorParamsAs1DForOutWhenUnconnected=off
  wires:
  Gain/1 -> Sum/2
  Sqrt/1 -> Out1/1
  Math Function/1 -> Sum/1
  Unit Delay/1 -> Gain/1
  Gain1/1 -> Unit Delay/1, Sqrt/1
  Sum/1 -> Gain1/1
  In1/1 -> Math Function/1

== system two_parallel_full_model_simscape/grid/instantaneus_power/rms4 ==
  In1 : Inport
  Gain : Gain  Gain=n10-1
  Gain1 : Gain  Gain=1/n10
  Math Function : Math  Operator=magnitude^2  SignedPower=on
  Sqrt : Sqrt
  Sum : Sum  Inputs=|++
  Unit Delay : UnitDelay  SampleTime=ts_afe  HasFrameUpgradeWarning=on
  Out1 : Outport  VectorParamsAs1DForOutWhenUnconnected=off
  wires:
  In1/1 -> Math Function/1
  Sum/1 -> Gain1/1
  Gain1/1 -> Sqrt/1, Unit Delay/1
  Unit Delay/1 -> Gain/1
  Math Function/1 -> Sum/1
  Sqrt/1 -> Out1/1
  Gain/1 -> Sum/2

== system two_parallel_full_model_simscape/grid/instantaneus_power/rms5 ==
  In1 : Inport
  Gain : Gain  Gain=n10-1
  Gain1 : Gain  Gain=1/n10
  Math Function : Math  Operator=magnitude^2  SignedPower=on
  Sqrt : Sqrt
  Sum : Sum  Inputs=|++
  Unit Delay : UnitDelay  SampleTime=ts_afe  HasFrameUpgradeWarning=on
  Out1 : Outport  VectorParamsAs1DForOutWhenUnconnected=off
  wires:
  Gain/1 -> Sum/2
  Sqrt/1 -> Out1/1
  Math Function/1 -> Sum/1
  Unit Delay/1 -> Gain/1
  Gain1/1 -> Unit Delay/1, Sqrt/1
  Sum/1 -> Gain1/1
  In1/1 -> Math Function/1

== system two_parallel_full_model_simscape/inverter_modA/single phase inverter/switch_1 ==
  Diode : fl_lib/Electrical/Electrical Elements/Diode  Vf=Vdon_diode V  Ron=Rdon_diode Ohm  Goff=1e-8 1/Ohm  i_specify=off  i_priority=None  i=0 A  i_nominal_specify=off  i_nominal_unit=A  i_nominal_value=1  v_specify=off  v_priority=None  v=0 V  v_nominal_specify=off  v_nominal_unit=V  v_nominal_value=1
  Switch : fl_lib/Electrical/Electrical Elements/Switch  R_closed=Ron Ohm  G_open=1e-8 1/Ohm  Threshold=7.5  i_specify=off  i_priority=None  i=0 A  i_nominal_specify=off  i_nominal_unit=A  i_nominal_value=1  v_specify=off  v_priority=None  v=0 V  v_nominal_specify=off  v_nominal_unit=V  v_nominal_value=1
  G : PMIOPort  Side=Left
  C : PMIOPort  Port=2  Side=Left
  E : PMIOPort  Port=3  Side=Right
  connections:
  Switch/RConn2 -- C/RConn1 -- Diode/RConn1
  Switch/RConn1 -- G/RConn1
  Switch/LConn1 -- E/RConn1 -- Diode/LConn1

== system two_parallel_full_model_simscape/inverter_modA/single phase inverter/switch_2 ==
  Diode : fl_lib/Electrical/Electrical Elements/Diode  Vf=Vdon_diode V  Ron=Rdon_diode Ohm  Goff=1e-8 1/Ohm  i_specify=off  i_priority=None  i=0 A  i_nominal_specify=off  i_nominal_unit=A  i_nominal_value=1  v_specify=off  v_priority=None  v=0 V  v_nominal_specify=off  v_nominal_unit=V  v_nominal_value=1
  Switch : fl_lib/Electrical/Electrical Elements/Switch  R_closed=Ron Ohm  G_open=1e-8 1/Ohm  Threshold=7.5  i_specify=off  i_priority=None  i=0 A  i_nominal_specify=off  i_nominal_unit=A  i_nominal_value=1  v_specify=off  v_priority=None  v=0 V  v_nominal_specify=off  v_nominal_unit=V  v_nominal_value=1
  G : PMIOPort  Side=Left
  C : PMIOPort  Port=2  Side=Left
  E : PMIOPort  Port=3  Side=Right
  connections:
  Diode/LConn1 -- E/RConn1 -- Switch/LConn1
  Switch/RConn1 -- G/RConn1
  Diode/RConn1 -- C/RConn1 -- Switch/RConn2

== system two_parallel_full_model_simscape/inverter_modA/single phase inverter/switch_3 ==
  Diode : fl_lib/Electrical/Electrical Elements/Diode  Vf=Vdon_diode V  Ron=Rdon_diode Ohm  Goff=1e-8 1/Ohm  i_specify=off  i_priority=None  i=0 A  i_nominal_specify=off  i_nominal_unit=A  i_nominal_value=1  v_specify=off  v_priority=None  v=0 V  v_nominal_specify=off  v_nominal_unit=V  v_nominal_value=1
  Switch : fl_lib/Electrical/Electrical Elements/Switch  R_closed=Ron Ohm  G_open=1e-8 1/Ohm  Threshold=7.5  i_specify=off  i_priority=None  i=0 A  i_nominal_specify=off  i_nominal_unit=A  i_nominal_value=1  v_specify=off  v_priority=None  v=0 V  v_nominal_specify=off  v_nominal_unit=V  v_nominal_value=1
  G : PMIOPort  Side=Left
  C : PMIOPort  Port=2  Side=Left
  E : PMIOPort  Port=3  Side=Right
  connections:
  Switch/RConn2 -- C/RConn1 -- Diode/RConn1
  Switch/RConn1 -- G/RConn1
  Switch/LConn1 -- E/RConn1 -- Diode/LConn1

== system two_parallel_full_model_simscape/inverter_modA/single phase inverter/switch_4 ==
  Diode : fl_lib/Electrical/Electrical Elements/Diode  Vf=Vdon_diode V  Ron=Rdon_diode Ohm  Goff=1e-8 1/Ohm  i_specify=off  i_priority=None  i=0 A  i_nominal_specify=off  i_nominal_unit=A  i_nominal_value=1  v_specify=off  v_priority=None  v=0 V  v_nominal_specify=off  v_nominal_unit=V  v_nominal_value=1
  Switch : fl_lib/Electrical/Electrical Elements/Switch  R_closed=Ron Ohm  G_open=1e-8 1/Ohm  Threshold=7.5  i_specify=off  i_priority=None  i=0 A  i_nominal_specify=off  i_nominal_unit=A  i_nominal_value=1  v_specify=off  v_priority=None  v=0 V  v_nominal_specify=off  v_nominal_unit=V  v_nominal_value=1
  G : PMIOPort  Side=Left
  C : PMIOPort  Port=2  Side=Left
  E : PMIOPort  Port=3  Side=Right
  connections:
  Diode/LConn1 -- E/RConn1 -- Switch/LConn1
  Switch/RConn1 -- G/RConn1
  Diode/RConn1 -- C/RConn1 -- Switch/RConn2

== system two_parallel_full_model_simscape/inverter_modA/single phase inverter control/acquisition_and_scaling_current ==
  in : Inport
  1/Ti5 : Gain  Gain=1/I_FS  SaturateOnIntegerOverflow=on  OutDataTypeStr=Inherit: Same as input  ParamDataTypeStr=Inherit: Same as input
  Unit Delay4 : UnitDelay  SampleTime=ts_inv  HasFrameUpgradeWarning=on
  Zero-Order Hold1 : ZeroOrderHold  SampleTime=ts_inv
  out : Outport
  wires:
  in/1 -> Zero-Order Hold1/1
  1/Ti5/1 -> Unit Delay4/1
  Zero-Order Hold1/1 -> 1/Ti5/1
  Unit Delay4/1 -> out/1

== system two_parallel_full_model_simscape/inverter_modA/single phase inverter control/acquisition_and_scaling_voltage ==
  in : Inport
  1/Ti1 : Gain  Gain=1/V_FS  SaturateOnIntegerOverflow=on  OutDataTypeStr=Inherit: Same as input  ParamDataTypeStr=Inherit: Same as input
  Unit Delay4 : UnitDelay  SampleTime=ts_inv  HasFrameUpgradeWarning=on
  Zero-Order Hold2 : ZeroOrderHold  SampleTime=ts_inv
  out : Outport
  wires:
  1/Ti1/1 -> Unit Delay4/1
  Zero-Order Hold2/1 -> 1/Ti1/1
  Unit Delay4/1 -> out/1
  in/1 -> Zero-Order Hold2/1

== system two_parallel_full_model_simscape/inverter_modA/single phase inverter control/alphabeta2dq ==
  note: va=V cos(wt)
      | vb=V cos(wt-2pi/3)
      | vc=V cos(wt+2pi/3)
  alpha : Inport
  beta : Inport  Port=2
  wt : Inport  Port=3
  Product{,1..3} (4 alike) : Product  RndMeth=Zero
  Sum : Sum
  Sum1 : Sum  Inputs=-+
  To Workspace1 : ToWorkspace  VariableName=id_pu_modA_sim  SampleTime=ts_inv
      settings: MaxDataPoints=Ns_inv
  To Workspace2 : ToWorkspace  VariableName=iq_pu_modA_sim  SampleTime=ts_inv
      settings: MaxDataPoints=Ns_inv
  Trigonometric Function : Trigonometry  Operator=cos
  Trigonometric Function1 : Trigonometry
  "d " : Outport  VectorParamsAs1DForOutWhenUnconnected=off
  "q " : Outport  Port=2  VectorParamsAs1DForOutWhenUnconnected=off
  wires:
  wt/1 -> Trigonometric Function1/1, Trigonometric Function/1
  Trigonometric Function/1 -> [cos]
  Trigonometric Function1/1 -> [sin]
  [cos] -> Product/1
  alpha/1 -> Product/2, Product2/2
  Product/1 -> Sum/1
  Product1/1 -> Sum/2
  [sin] -> Product1/1
  beta/1 -> Product1/2, Product3/2
  Sum/1 -> To Workspace1/1, "d "/1
  [sin] -> Product2/1
  Product2/1 -> Sum1/1
  Product3/1 -> Sum1/2
  [cos] -> Product3/1
  Sum1/1 -> To Workspace2/1, "q "/1

== system two_parallel_full_model_simscape/inverter_modA/single phase inverter control/dq2alphabeta ==
  d : Inport
  q : Inport  Port=2
  wt : Inport  Port=3
  Product{,1..3} (4 alike) : Product  RndMeth=Zero
  Sum : Sum  Inputs=+-
  Sum1 : Sum
  Trigonometric Function : Trigonometry  Operator=cos
  Trigonometric Function1 : Trigonometry
  alpha : Outport  VectorParamsAs1DForOutWhenUnconnected=off
  wires:
  [cos] -> Product3/1
  Product3/1 -> Sum1/2
  Product2/1 -> Sum1/1
  [sin] -> Product2/1
  Sum/1 -> alpha/1
  q/1 -> Product3/2, Product1/2
  [sin] -> Product1/1
  Product1/1 -> Sum/2
  Product/1 -> Sum/1
  d/1 -> Product2/2, Product/2
  [cos] -> Product/1
  Trigonometric Function1/1 -> [sin]
  Trigonometric Function/1 -> [cos]
  wt/1 -> Trigonometric Function/1, Trigonometric Function1/1

== system two_parallel_full_model_simscape/inverter_modA/single phase inverter control/pi_d ==
  id_tilde : Inport
  1/Ti : Gain  Gain=kp_i_inv  SaturateOnIntegerOverflow=on  OutDataTypeStr=Inherit: Same as input  ParamDataTypeStr=Inherit: Same as input
  Sum1 : Sum  Inputs=+++  SaturateOnIntegerOverflow=on
  Sum3 : Sum  Inputs=-+  SaturateOnIntegerOverflow=on
  To Workspace3 : ToWorkspace  VariableName=id_ctrl_out_modA_sim  SampleTime=ts_inv
      settings: MaxDataPoints=Ns_inv
  Unit Delay4 : UnitDelay  SampleTime=ts_inv  HasFrameUpgradeWarning=on
  kp2 : Gain  Gain=ki_i_inv*ts_inv  SaturateOnIntegerOverflow=on  OutDataTypeStr=Inherit: Same as input  ParamDataTypeStr=Inherit: Same as input
  ud_out_lim : Saturate  UpperLimit=1  LowerLimit=-1
  "ud_out_lim " : Saturate  UpperLimit=1  LowerLimit=-1
  Vd_out : Outport  VectorParamsAs1DForOutWhenUnconnected=off
  wires:
  id_tilde/1 -> kp2/1, 1/Ti/1
  Sum1/1 -> ud_out_lim/1
  kp2/1 -> Sum1/2
  1/Ti/1 -> Sum1/1, Sum3/1
  Unit Delay4/1 -> Sum1/3
  Sum3/1 -> Unit Delay4/1
  ud_out_lim/1 -> Sum3/2, "ud_out_lim "/1
  "ud_out_lim "/1 -> To Workspace3/1, Vd_out/1

== system two_parallel_full_model_simscape/inverter_modA/single phase inverter control/pi_q ==
  iq_tilde : Inport
  1/Ti : Gain  Gain=kp_i_inv  SaturateOnIntegerOverflow=on  OutDataTypeStr=Inherit: Same as input  ParamDataTypeStr=Inherit: Same as input
  Sum1 : Sum  Inputs=+++  SaturateOnIntegerOverflow=on
  Sum3 : Sum  Inputs=-+  SaturateOnIntegerOverflow=on
  To Workspace3 : ToWorkspace  VariableName=iq_ctrl_out_modA_sim  SampleTime=ts_inv
      settings: MaxDataPoints=Ns_inv
  Unit Delay4 : UnitDelay  SampleTime=ts_inv  HasFrameUpgradeWarning=on
  kp2 : Gain  Gain=ki_i_inv*ts_inv  SaturateOnIntegerOverflow=on  OutDataTypeStr=Inherit: Same as input  ParamDataTypeStr=Inherit: Same as input
  ud_out_lim : Saturate  UpperLimit=1  LowerLimit=-1
  "uq_out_lim " : Saturate  UpperLimit=1  LowerLimit=-1
  Vd_out : Outport  VectorParamsAs1DForOutWhenUnconnected=off
  wires:
  "uq_out_lim "/1 -> Vd_out/1, To Workspace3/1
  ud_out_lim/1 -> "uq_out_lim "/1, Sum3/2
  Sum3/1 -> Unit Delay4/1
  Unit Delay4/1 -> Sum1/3
  1/Ti/1 -> Sum3/1, Sum1/1
  kp2/1 -> Sum1/2
  Sum1/1 -> ud_out_lim/1
  iq_tilde/1 -> 1/Ti/1, kp2/1

== system two_parallel_full_model_simscape/inverter_modA/single phase inverter control/pi_v ==
  e : Inport
  1/Ti : Gain  Gain=kp_v_inv  SaturateOnIntegerOverflow=on  OutDataTypeStr=Inherit: Same as input  ParamDataTypeStr=Inherit: Same as input
  Sum1 : Sum  Inputs=+++  SaturateOnIntegerOverflow=on
  Sum3 : Sum  Inputs=-+  SaturateOnIntegerOverflow=on
  To Workspace3 : ToWorkspace  VariableName=v_ctrl_out_modA_sim  SampleTime=ts_inv
      settings: MaxDataPoints=Ns_inv
  Unit Delay4 : UnitDelay  SampleTime=ts_inv  HasFrameUpgradeWarning=on
  i_out_lim : Saturate  UpperLimit=0.869565217391304  LowerLimit=0
  kp2 : Gain  Gain=ki_v_inv*ts_inv  SaturateOnIntegerOverflow=on  OutDataTypeStr=Inherit: Same as input  ParamDataTypeStr=Inherit: Same as input
  i_ref_internal : Outport  VectorParamsAs1DForOutWhenUnconnected=off
  wires:
  i_out_lim/1 -> i_ref_internal/1, To Workspace3/1, Sum3/2
  Sum3/1 -> Unit Delay4/1
  Unit Delay4/1 -> Sum1/3
  1/Ti/1 -> Sum3/1, Sum1/1
  kp2/1 -> Sum1/2
  Sum1/1 -> i_out_lim/1
  e/1 -> kp2/1, 1/Ti/1

== system two_parallel_full_model_simscape/inverter_modA/single phase inverter control/pwm ==
  vout : Inport
  Constant : Constant  Value=0
  Constant1 : Constant
  Constant2 : Constant
  Constant3 : Constant
  Gain1 : Gain  Gain=1/2
  Gain2 : Gain
  Gain3 : Gain  Gain=1/2
  Gain4 : Gain  Gain=-1
  PWM generator 1 : Subsystem  mask{f=fPWM_INV, m_up=1, m_low=0, dead_time=0, pos_cmd_gate=15, neg_cmd_gate=-10, polarity=-1}
      mask prompts: f "Frequency (Hz)"; m_up "Max Input Modulation Value"; m_low "Min Input Modulation Value"; dead_time "Dead Time (s)"; pos_cmd_gate "Positive Gate Voltage (V)"; neg_cmd_gate "Negative Gate Voltage (V)"; polarity "Polarity (pu)"
  PWM generator 2 : Subsystem  mask{f=fPWM_INV, m_up=1, m_low=0, dead_time=0, pos_cmd_gate=15, neg_cmd_gate=-10, polarity=-1}
      mask prompts: f "Frequency (Hz)"; m_up "Max Input Modulation Value"; m_low "Min Input Modulation Value"; dead_time "Dead Time (s)"; pos_cmd_gate "Positive Gate Voltage (V)"; neg_cmd_gate "Negative Gate Voltage (V)"; polarity "Polarity (pu)"
  Sum : Sum  Inputs=|++
  Sum1 : Sum  Inputs=|++
  m1_top : Outport
  m1_bottom : Outport  Port=2
  m2_top : Outport  Port=3
  m2_bottom : Outport  Port=4
  wires:
  PWM generator 1/1(m1) -> m1_top/1  "gate_cmd_Q1"
  PWM generator 1/2(m2) -> m1_bottom/1  "gate_cmd_Q2"
  PWM generator 2/2(m2) -> m2_bottom/1  "gate_cmd_Q2"
  PWM generator 2/1(m1) -> m2_top/1  "gate_cmd_Q1"
  Constant/1 -> PWM generator 2/2(phase), PWM generator 1/2(phase)
  Constant1/1 -> PWM generator 2/3(polarity_input), PWM generator 1/3(polarity_input)
  Gain2/1 -> Sum/1
  Sum/1 -> Gain1/1
  Constant2/1 -> Sum/2
  Gain1/1 -> PWM generator 1/1(m_index)
  Constant3/1 -> Sum1/2
  Sum1/1 -> Gain3/1
  Gain4/1 -> Sum1/1
  Gain3/1 -> PWM generator 2/1(m_index)
  vout/1 -> Gain4/1, Gain2/1

== system two_parallel_full_model_simscape/inverter_modB/single phase inverter/switch_1 ==
  Diode : fl_lib/Electrical/Electrical Elements/Diode  Vf=Vdon_diode V  Ron=Rdon_diode Ohm  Goff=1e-8 1/Ohm  i_specify=off  i_priority=None  i=0 A  i_nominal_specify=off  i_nominal_unit=A  i_nominal_value=1  v_specify=off  v_priority=None  v=0 V  v_nominal_specify=off  v_nominal_unit=V  v_nominal_value=1
  Switch : fl_lib/Electrical/Electrical Elements/Switch  R_closed=Ron Ohm  G_open=1e-8 1/Ohm  Threshold=7.5  i_specify=off  i_priority=None  i=0 A  i_nominal_specify=off  i_nominal_unit=A  i_nominal_value=1  v_specify=off  v_priority=None  v=0 V  v_nominal_specify=off  v_nominal_unit=V  v_nominal_value=1
  G : PMIOPort  Side=Left
  C : PMIOPort  Port=2  Side=Left
  E : PMIOPort  Port=3  Side=Right
  connections:
  Diode/LConn1 -- E/RConn1 -- Switch/LConn1
  Switch/RConn1 -- G/RConn1
  Diode/RConn1 -- C/RConn1 -- Switch/RConn2

== system two_parallel_full_model_simscape/inverter_modB/single phase inverter/switch_2 ==
  Diode : fl_lib/Electrical/Electrical Elements/Diode  Vf=Vdon_diode V  Ron=Rdon_diode Ohm  Goff=1e-8 1/Ohm  i_specify=off  i_priority=None  i=0 A  i_nominal_specify=off  i_nominal_unit=A  i_nominal_value=1  v_specify=off  v_priority=None  v=0 V  v_nominal_specify=off  v_nominal_unit=V  v_nominal_value=1
  Switch : fl_lib/Electrical/Electrical Elements/Switch  R_closed=Ron Ohm  G_open=1e-8 1/Ohm  Threshold=7.5  i_specify=off  i_priority=None  i=0 A  i_nominal_specify=off  i_nominal_unit=A  i_nominal_value=1  v_specify=off  v_priority=None  v=0 V  v_nominal_specify=off  v_nominal_unit=V  v_nominal_value=1
  G : PMIOPort  Side=Left
  C : PMIOPort  Port=2  Side=Left
  E : PMIOPort  Port=3  Side=Right
  connections:
  Switch/RConn2 -- C/RConn1 -- Diode/RConn1
  Switch/RConn1 -- G/RConn1
  Switch/LConn1 -- E/RConn1 -- Diode/LConn1
